simulink model "large_scale_autosar_swc_expfcns"  (R2021a)
settings: Solver=FixedStepDiscrete  StartTime=0.0  StopTime=20  FixedStep=1  MaxStep=.0001  RelTol=1e-3  EnableMultiTasking=on
undefined symbols (not defined in the file): DiscIntNeverNeededParam
(part 1 of 3)
settings Model: ExtModeAutoUpdateStatusClock=off  Creator=The MathWorks, Inc.  LastModifiedBy=ASUS
settings SolverCC: AlgebraicLoopSolver=TrustRegion
settings DataIOCC: LimitDataPoints=on  SaveFormat=Array  SaveOutput=off  SaveTime=off  ReturnWorkspaceOutputs=off
settings OptimizationCC: DefaultParameterBehavior=Inlined  InlineInvariantSignals=on  EnhancedBackFolding=on  ExpressionDepthLimit=2147483647  StateBitsets=on  DataBitsets=on  ZeroExternalMemoryAtStartup=off  ZeroInternalMemoryAtStartup=off  NoFixptDivByZeroProtection=on  EfficientFloat2IntCast=on  EfficientMapNaN2IntZero=off  LifeSpan=1  BufferReusableBoundary=off  EfficientTunableParamExpr=on
settings DebuggingCC: SigSpecEnsureSampleTimeMsg=none  BusObjectLabelMismatch=none  AllowSymbolicDim=off  StateNameClashWarn=warning  PregeneratedLibrarySubsystemCodeDiagnostic=none  StrictBusMsg=ErrorOnBusTreatedAsVector  SFUnexpectedBacktrackingDiag=warning  SFNoUnconditionalDefaultTransitionDiag=warning  SFExecutionAtInitializationDiag=none  SFMachineParentedDataDiag=warning  ArithmeticOperatorsInVariantConditions=warning
settings HardwareCC: ProdLongLongMode=on  TargetIntDivRoundTo=Zero  TargetEndianess=LittleEndian  TargetHWDeviceType=Generic->32-bit Embedded Processor
settings ModelReferenceCC: ModelReferenceNumInstancesAllowed=Single  PropagateSignalLabelsOutOfModel=off
settings SFSimCC: SimUseLocalCustomCode=off  SimParseCustomCode=off  CustomCodeUndefinedFunction=UseInterfaceOnly
settings RTWCC: Description=AUTOSAR  SystemTargetFile=autosar.tlc  GenCodeOnly=on  TemplateMakefile=ert_default_tmf  GenerateReport=on  RTWVerbose=off  RTWUseLocalCustomCode=off  IncludeHyperlinkInReport=on  LaunchReport=on  PortableWordSizes=on
settings CodeAppCC: ForceParamTrailComments=on  IgnoreCustomStorageClasses=off  IgnoreTestpoints=on  SimulinkDataObjDesc=on  CustomSymbolStrGlobalVar=rt$N$M  CustomSymbolStrType=$N$M  CustomSymbolStrFcn=$N$M$F  CustomSymbolStrMacro=$N$M  InsertBlockDesc=on  StateflowObjectComments=on  InternalIdentifier=Classic
settings STFCustomTargetCC: UtilityFuncGeneration=Shared location  ParMdlRefBuildCompliant=on  CompOptLevelCompliant=on  IncludeMdlTerminateFcn=off  CombineOutputUpdateFcns=on  SuppressErrorStatus=on  ERTCustomFileBanners=on  SupportNonFinite=off  SupportComplex=off  SupportContinuousTime=off  SupportNonInlinedSFcns=off  RemoveResetFunc=on  MATLABClassNameForMDSCustomization=Simulink.SoftwareTarget.ERTCustomization  CPPClassGenCompliant=on  AutosarCompliant=on  GRTInterface=off  LookupTableObjectStructAxisOrder=2,1,3,4,...  LUTObjectStructOrderEvenSpacing=Size,Table,Breakpoints  SystemTargetFile=autosar.tlc
settings ERTTargetCC: UtilityFuncGeneration=Shared location  MultiwordLength=2048  ConcurrentExecutionCompliant=off  IncludeMdlTerminateFcn=off  SuppressErrorStatus=on  SupportNonFinite=off  SupportComplex=off  ModelStepFunctionPrototypeControlCompliant=off  AutosarCompliant=on  LookupTableObjectStructAxisOrder=2,1,3,4,...  LUTObjectStructOrderEvenSpacing=Size,Table,Breakpoints  ExtModeMexFile=noextcomm  InlinedParameterPlacement=NonHierarchical  ERTCustomFileTemplate=example_file_process.tlc  ERTFilePackagingFormat=CompactWithDataFile  ConvertIfToSwitch=off  SuppressUnreachableDefaultCases=off
settings ConfigComp: CovMetricSettings=dw  CovSaveCumulativeToWorkspaceVar=on  CovSaveSingleToWorkspaceVar=on  CovExternalEMLEnable=off

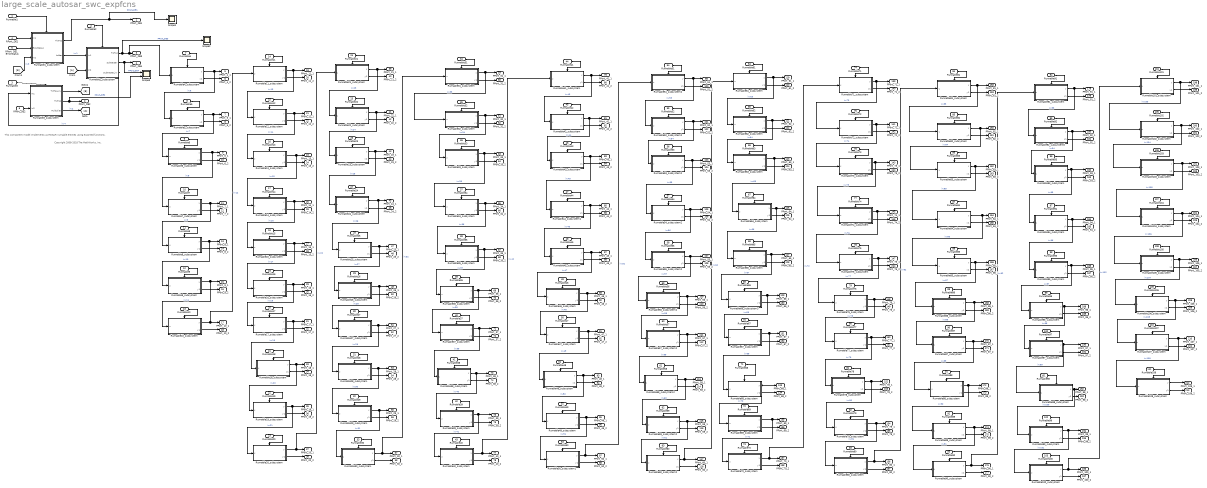
== system large_scale_autosar_swc_expfcns ==
  note: This component model implements AUTOSAR runnable entities using exported functions.
  note: Copyright 2008-2018 The MathWorks, Inc.
  Runnable1 : Inport  PortDimensions=1  SampleTime=1  OutputFunctionCall=on
  Runnable2 : Inport  Port=2  PortDimensions=1  SampleTime=1  OutputFunctionCall=on
  Runnable3 : Inport  Port=3  PortDimensions=1  SampleTime=10  OutputFunctionCall=on
  RPort_DE1 : Inport  Port=4  OutDataTypeStr=double  PortDimensions=1
  RPort_DE1_ErrorStatus : Inport  Port=5  OutDataTypeStr=uint8  PortDimensions=1
  RPort_DE2 : Inport  Port=6  OutDataTypeStr=double  PortDimensions=2
  Runnable4 : Inport  Port=7  PortDimensions=1  SampleTime=1  OutputFunctionCall=on
  Runnable5 : Inport  Port=8  PortDimensions=1  SampleTime=1  OutputFunctionCall=on
  Runnable6 : Inport  Port=9  PortDimensions=1  SampleTime=1  OutputFunctionCall=on
  Runnable7 : Inport  Port=10  PortDimensions=1  SampleTime=1  OutputFunctionCall=on
  Runnable8 : Inport  Port=11  PortDimensions=1  SampleTime=1  OutputFunctionCall=on
  Runnable9 : Inport  Port=12  PortDimensions=1  SampleTime=1  OutputFunctionCall=on
  Runnable10 : Inport  Port=13  PortDimensions=1  SampleTime=1  OutputFunctionCall=on
  Runnable11 : Inport  Port=14  PortDimensions=1  SampleTime=1  OutputFunctionCall=on
  Runnable12 : Inport  Port=15  PortDimensions=1  SampleTime=1  OutputFunctionCall=on
  Runnable13 : Inport  Port=16  PortDimensions=1  SampleTime=1  OutputFunctionCall=on
  Runnable14 : Inport  Port=17  PortDimensions=1  SampleTime=1  OutputFunctionCall=on
  Runnable15 : Inport  Port=18  PortDimensions=1  SampleTime=1  OutputFunctionCall=on
  Runnable16 : Inport  Port=19  PortDimensions=1  SampleTime=1  OutputFunctionCall=on
  Runnable17 : Inport  Port=20  PortDimensions=1  SampleTime=1  OutputFunctionCall=on
  Runnable18 : Inport  Port=21  PortDimensions=1  SampleTime=1  OutputFunctionCall=on
  Runnable19 : Inport  Port=22  PortDimensions=1  SampleTime=1  OutputFunctionCall=on
  Runnable20 : Inport  Port=23  PortDimensions=1  SampleTime=1  OutputFunctionCall=on
  Runnable21 : Inport  Port=24  PortDimensions=1  SampleTime=1  OutputFunctionCall=on
  Runnable22 : Inport  Port=25  PortDimensions=1  SampleTime=1  OutputFunctionCall=on
  Runnable23 : Inport  Port=26  PortDimensions=1  SampleTime=1  OutputFunctionCall=on
  Runnable24 : Inport  Port=27  PortDimensions=1  SampleTime=1  OutputFunctionCall=on
  Runnable25 : Inport  Port=28  PortDimensions=1  SampleTime=1  OutputFunctionCall=on
  Runnable26 : Inport  Port=29  PortDimensions=1  SampleTime=1  OutputFunctionCall=on
  Runnable27 : Inport  Port=30  PortDimensions=1  SampleTime=1  OutputFunctionCall=on
  Runnable28 : Inport  Port=31  PortDimensions=1  SampleTime=1  OutputFunctionCall=on
  Runnable29 : Inport  Port=32  PortDimensions=1  SampleTime=1  OutputFunctionCall=on
  Runnable30 : Inport  Port=33  PortDimensions=1  SampleTime=1  OutputFunctionCall=on
  Runnable31 : Inport  Port=34  PortDimensions=1  SampleTime=1  OutputFunctionCall=on
  Runnable32 : Inport  Port=35  PortDimensions=1  SampleTime=1  OutputFunctionCall=on
  Runnable33 : Inport  Port=36  PortDimensions=1  SampleTime=1  OutputFunctionCall=on
  Runnable34 : Inport  Port=37  PortDimensions=1  SampleTime=1  OutputFunctionCall=on
  Runnable35 : Inport  Port=38  PortDimensions=1  SampleTime=1  OutputFunctionCall=on
  Runnable36 : Inport  Port=39  PortDimensions=1  SampleTime=1  OutputFunctionCall=on
  Runnable37 : Inport  Port=40  PortDimensions=1  SampleTime=1  OutputFunctionCall=on
  Runnable38 : Inport  Port=41  PortDimensions=1  SampleTime=1  OutputFunctionCall=on
  Runnable39 : Inport  Port=42  PortDimensions=1  SampleTime=1  OutputFunctionCall=on
  Runnable40 : Inport  Port=43  PortDimensions=1  SampleTime=1  OutputFunctionCall=on
  Runnable41 : Inport  Port=44  PortDimensions=1  SampleTime=1  OutputFunctionCall=on
  Runnable42 : Inport  Port=45  PortDimensions=1  SampleTime=1  OutputFunctionCall=on
  Runnable43 : Inport  Port=46  PortDimensions=1  SampleTime=1  OutputFunctionCall=on
  Runnable44 : Inport  Port=47  PortDimensions=1  SampleTime=1  OutputFunctionCall=on
  Runnable45 : Inport  Port=48  PortDimensions=1  SampleTime=1  OutputFunctionCall=on
  Runnable46 : Inport  Port=49  PortDimensions=1  SampleTime=1  OutputFunctionCall=on
  Runnable47 : Inport  Port=50  PortDimensions=1  SampleTime=1  OutputFunctionCall=on
  Runnable48 : Inport  Port=51  PortDimensions=1  SampleTime=1  OutputFunctionCall=on
  Runnable49 : Inport  Port=52  PortDimensions=1  SampleTime=1  OutputFunctionCall=on
  Runnable50 : Inport  Port=53  PortDimensions=1  SampleTime=1  OutputFunctionCall=on
  Runnable51 : Inport  Port=54  PortDimensions=1  SampleTime=1  OutputFunctionCall=on
  Runnable52 : Inport  Port=55  PortDimensions=1  SampleTime=1  OutputFunctionCall=on
  Runnable53 : Inport  Port=56  PortDimensions=1  SampleTime=1  OutputFunctionCall=on
  Runnable54 : Inport  Port=57  PortDimensions=1  SampleTime=1  OutputFunctionCall=on
  Runnable55 : Inport  Port=58  PortDimensions=1  SampleTime=1  OutputFunctionCall=on
  Runnable56 : Inport  Port=59  PortDimensions=1  SampleTime=1  OutputFunctionCall=on
  Runnable57 : Inport  Port=60  PortDimensions=1  SampleTime=1  OutputFunctionCall=on
  Runnable58 : Inport  Port=61  PortDimensions=1  SampleTime=1  OutputFunctionCall=on
  Runnable59 : Inport  Port=62  PortDimensions=1  SampleTime=1  OutputFunctionCall=on
  Runnable60 : Inport  Port=63  PortDimensions=1  SampleTime=1  OutputFunctionCall=on
  Runnable61 : Inport  Port=64  PortDimensions=1  SampleTime=1  OutputFunctionCall=on
  Runnable62 : Inport  Port=65  PortDimensions=1  SampleTime=1  OutputFunctionCall=on
  Runnable63 : Inport  Port=66  PortDimensions=1  SampleTime=1  OutputFunctionCall=on
  Runnable64 : Inport  Port=67  PortDimensions=1  SampleTime=1  OutputFunctionCall=on
  Runnable65 : Inport  Port=68  PortDimensions=1  SampleTime=1  OutputFunctionCall=on
  Runnable66 : Inport  Port=69  PortDimensions=1  SampleTime=1  OutputFunctionCall=on
  Runnable67 : Inport  Port=70  PortDimensions=1  SampleTime=1  OutputFunctionCall=on
  Runnable68 : Inport  Port=71  PortDimensions=1  SampleTime=1  OutputFunctionCall=on
  Runnable69 : Inport  Port=72  PortDimensions=1  SampleTime=1  OutputFunctionCall=on
  Runnable70 : Inport  Port=73  PortDimensions=1  SampleTime=1  OutputFunctionCall=on
  Runnable71 : Inport  Port=74  PortDimensions=1  SampleTime=1  OutputFunctionCall=on
  Runnable72 : Inport  Port=75  PortDimensions=1  SampleTime=1  OutputFunctionCall=on
  Runnable73 : Inport  Port=76  PortDimensions=1  SampleTime=1  OutputFunctionCall=on
  Runnable74 : Inport  Port=77  PortDimensions=1  SampleTime=1  OutputFunctionCall=on
  Runnable75 : Inport  Port=78  PortDimensions=1  SampleTime=1  OutputFunctionCall=on
  Runnable76 : Inport  Port=79  PortDimensions=1  SampleTime=1  OutputFunctionCall=on
  Runnable77 : Inport  Port=80  PortDimensions=1  SampleTime=1  OutputFunctionCall=on
  Runnable78 : Inport  Port=81  PortDimensions=1  SampleTime=1  OutputFunctionCall=on
  Runnable79 : Inport  Port=82  PortDimensions=1  SampleTime=1  OutputFunctionCall=on
  Runnable80 : Inport  Port=83  PortDimensions=1  SampleTime=1  OutputFunctionCall=on
  Runnable81 : Inport  Port=84  PortDimensions=1  SampleTime=1  OutputFunctionCall=on
  Runnable82 : Inport  Port=85  PortDimensions=1  SampleTime=1  OutputFunctionCall=on
  Runnable83 : Inport  Port=86  PortDimensions=1  SampleTime=1  OutputFunctionCall=on
  Runnable84 : Inport  Port=87  PortDimensions=1  SampleTime=1  OutputFunctionCall=on
  Runnable85 : Inport  Port=88  PortDimensions=1  SampleTime=1  OutputFunctionCall=on
  Runnable86 : Inport  Port=89  PortDimensions=1  SampleTime=1  OutputFunctionCall=on
  Runnable87 : Inport  Port=90  PortDimensions=1  SampleTime=1  OutputFunctionCall=on
  Runnable88 : Inport  Port=91  PortDimensions=1  SampleTime=1  OutputFunctionCall=on
  Runnable89 : Inport  Port=92  PortDimensions=1  SampleTime=1  OutputFunctionCall=on
  Runnable90 : Inport  Port=93  PortDimensions=1  SampleTime=1  OutputFunctionCall=on
  Runnable91 : Inport  Port=94  PortDimensions=1  SampleTime=1  OutputFunctionCall=on
  Runnable92 : Inport  Port=95  PortDimensions=1  SampleTime=1  OutputFunctionCall=on
  Runnable93 : Inport  Port=96  PortDimensions=1  SampleTime=1  OutputFunctionCall=on
  Runnable94 : Inport  Port=97  PortDimensions=1  SampleTime=1  OutputFunctionCall=on
  Runnable95 : Inport  Port=98  PortDimensions=1  SampleTime=1  OutputFunctionCall=on
  Runnable96 : Inport  Port=99  PortDimensions=1  SampleTime=1  OutputFunctionCall=on
  Runnable97 : Inport  Port=100  PortDimensions=1  SampleTime=1  OutputFunctionCall=on
  Runnable98 : Inport  Port=101  PortDimensions=1  SampleTime=1  OutputFunctionCall=on
  Runnable99 : Inport  Port=102  PortDimensions=1  SampleTime=1  OutputFunctionCall=on
  Runnable100 : Inport  Port=103  PortDimensions=1  SampleTime=1  OutputFunctionCall=on
  Runnable101 : Inport  Port=104  PortDimensions=1  SampleTime=1  OutputFunctionCall=on
  Runnable102 : Inport  Port=105  PortDimensions=1  SampleTime=1  OutputFunctionCall=on
  Runnable103 : Inport  Port=106  PortDimensions=1  SampleTime=1  OutputFunctionCall=on
  Runnable104 : Inport  Port=107  PortDimensions=1  SampleTime=1  OutputFunctionCall=on
  Runnable105 : Inport  Port=108  PortDimensions=1  SampleTime=1  OutputFunctionCall=on
  Runnable106 : Inport  Port=109  PortDimensions=1  SampleTime=1  OutputFunctionCall=on
  Runnable107 : Inport  Port=110  PortDimensions=1  SampleTime=1  OutputFunctionCall=on
  Runnable108 : Inport  Port=111  PortDimensions=1  SampleTime=1  OutputFunctionCall=on
  Runnable100_subsystem : Subsystem  TreatAsAtomicUnit=on  RTWFcnName=foo
  Runnable101_subsystem : Subsystem  TreatAsAtomicUnit=on  RTWFcnName=foo
  Runnable102_subsystem : Subsystem  TreatAsAtomicUnit=on  RTWFcnName=foo
  Runnable103_subsystem : Subsystem  TreatAsAtomicUnit=on  RTWFcnName=foo
  Runnable104_subsystem : Subsystem  TreatAsAtomicUnit=on  RTWFcnName=foo
  Runnable105_subsystem : Subsystem  TreatAsAtomicUnit=on  RTWFcnName=foo
  Runnable106_subsystem : Subsystem  TreatAsAtomicUnit=on  RTWFcnName=foo
  Runnable107_subsystem : Subsystem  TreatAsAtomicUnit=on  RTWFcnName=foo
  Runnable108_subsystem : Subsystem  TreatAsAtomicUnit=on  RTWFcnName=foo
  Runnable10_subsystem : Subsystem  TreatAsAtomicUnit=on  RTWFcnName=foo
  Runnable11_subsystem : Subsystem  TreatAsAtomicUnit=on  RTWFcnName=foo
  Runnable12_subsystem : Subsystem  TreatAsAtomicUnit=on  RTWFcnName=foo
  Runnable13_subsystem : Subsystem  TreatAsAtomicUnit=on  RTWFcnName=foo
  Runnable14_subsystem : Subsystem  TreatAsAtomicUnit=on  RTWFcnName=foo
  Runnable15_subsystem : Subsystem  TreatAsAtomicUnit=on  RTWFcnName=foo
  Runnable16_subsystem : Subsystem  TreatAsAtomicUnit=on  RTWFcnName=foo
  Runnable17_subsystem : Subsystem  TreatAsAtomicUnit=on  RTWFcnName=foo
  Runnable18_subsystem : Subsystem  TreatAsAtomicUnit=on  RTWFcnName=foo
  Runnable19_subsystem : Subsystem  TreatAsAtomicUnit=on  RTWFcnName=foo
  Runnable1_subsystem : Subsystem  TreatAsAtomicUnit=on  RTWFcnName=foo
  Runnable20_subsystem : Subsystem  TreatAsAtomicUnit=on  RTWFcnName=foo
  Runnable21_subsystem : Subsystem  TreatAsAtomicUnit=on  RTWFcnName=foo
  Runnable22_subsystem : Subsystem  TreatAsAtomicUnit=on  RTWFcnName=foo
  Runnable23_subsystem : Subsystem  TreatAsAtomicUnit=on  RTWFcnName=foo
  Runnable24_subsystem : Subsystem  TreatAsAtomicUnit=on  RTWFcnName=foo
  Runnable25_subsystem : Subsystem  TreatAsAtomicUnit=on  RTWFcnName=foo
  Runnable26_subsystem : Subsystem  TreatAsAtomicUnit=on  RTWFcnName=foo
  Runnable27_subsystem : Subsystem  TreatAsAtomicUnit=on  RTWFcnName=foo
  Runnable28_subsystem : Subsystem  TreatAsAtomicUnit=on  RTWFcnName=foo
  Runnable29_subsystem : Subsystem  TreatAsAtomicUnit=on  RTWFcnName=foo
  Runnable2_subsystem : Subsystem  TreatAsAtomicUnit=on  RTWFcnName=foo
  Runnable30_subsystem : Subsystem  TreatAsAtomicUnit=on  RTWFcnName=foo
  Runnable31_subsystem : Subsystem  TreatAsAtomicUnit=on  RTWFcnName=foo
  Runnable32_subsystem : Subsystem  TreatAsAtomicUnit=on  RTWFcnName=foo
  Runnable33_subsystem : Subsystem  TreatAsAtomicUnit=on  RTWFcnName=foo
  Runnable34_subsystem : Subsystem  TreatAsAtomicUnit=on  RTWFcnName=foo
  Runnable35_subsystem : Subsystem  TreatAsAtomicUnit=on  RTWFcnName=foo
  Runnable36_subsystem : Subsystem  TreatAsAtomicUnit=on  RTWFcnName=foo
  Runnable37_subsystem : Subsystem  TreatAsAtomicUnit=on  RTWFcnName=foo
  Runnable38_subsystem : Subsystem  TreatAsAtomicUnit=on  RTWFcnName=foo
  Runnable39_subsystem : Subsystem  TreatAsAtomicUnit=on  RTWFcnName=foo
  Runnable3_subsystem : Subsystem  TreatAsAtomicUnit=on  RTWFcnName=foo
  Runnable40_subsystem : Subsystem  TreatAsAtomicUnit=on  RTWFcnName=foo
  Runnable41_subsystem : Subsystem  TreatAsAtomicUnit=on  RTWFcnName=foo
  Runnable42_subsystem : Subsystem  TreatAsAtomicUnit=on  RTWFcnName=foo
  Runnable43_subsystem : Subsystem  TreatAsAtomicUnit=on  RTWFcnName=foo
  Runnable44_subsystem1 : Subsystem  TreatAsAtomicUnit=on  RTWFcnName=foo
  Runnable45_subsystem : Subsystem  TreatAsAtomicUnit=on  RTWFcnName=foo
  Runnable46_subsystem : Subsystem  TreatAsAtomicUnit=on  RTWFcnName=foo
  Runnable47_subsystem : Subsystem  TreatAsAtomicUnit=on  RTWFcnName=foo
  Runnable48_subsystem : Subsystem  TreatAsAtomicUnit=on  RTWFcnName=foo
  Runnable49_subsystem : Subsystem  TreatAsAtomicUnit=on  RTWFcnName=foo
  Runnable4_subsystem : Subsystem  TreatAsAtomicUnit=on  RTWFcnName=foo
  Runnable50_subsystem1 : Subsystem  TreatAsAtomicUnit=on  RTWFcnName=foo
  Runnable51_subsystem2 : Subsystem  TreatAsAtomicUnit=on  RTWFcnName=foo
  Runnable52_subsystem2 : Subsystem  TreatAsAtomicUnit=on  RTWFcnName=foo
  Runnable53_subsystem2 : Subsystem  TreatAsAtomicUnit=on  RTWFcnName=foo
  Runnable54_subsystem2 : Subsystem  TreatAsAtomicUnit=on  RTWFcnName=foo
  Runnable55_subsystem2 : Subsystem  TreatAsAtomicUnit=on  RTWFcnName=foo
  Runnable56_subsystem2 : Subsystem  TreatAsAtomicUnit=on  RTWFcnName=foo
  Runnable57_subsystem2 : Subsystem  TreatAsAtomicUnit=on  RTWFcnName=foo
  Runnable58_subsystem2 : Subsystem  TreatAsAtomicUnit=on  RTWFcnName=foo
  Runnable59_subsystem2 : Subsystem  TreatAsAtomicUnit=on  RTWFcnName=foo
  Runnable5_subsystem : Subsystem  TreatAsAtomicUnit=on  RTWFcnName=foo
  Runnable60_subsystem2 : Subsystem  TreatAsAtomicUnit=on  RTWFcnName=foo
  Runnable61_subsystem : Subsystem  TreatAsAtomicUnit=on  RTWFcnName=foo
  Runnable62_subsystem : Subsystem  TreatAsAtomicUnit=on  RTWFcnName=foo
  Runnable63_subsystem : Subsystem  TreatAsAtomicUnit=on  RTWFcnName=foo
  Runnable64_subsystem : Subsystem  TreatAsAtomicUnit=on  RTWFcnName=foo
  Runnable65_subsystem : Subsystem  TreatAsAtomicUnit=on  RTWFcnName=foo
  Runnable66_subsystem3 : Subsystem  TreatAsAtomicUnit=on  RTWFcnName=foo
  Runnable67_subsystem : Subsystem  TreatAsAtomicUnit=on  RTWFcnName=foo
  Runnable68_subsystem : Subsystem  TreatAsAtomicUnit=on  RTWFcnName=foo
  Runnable69_subsystem : Subsystem  TreatAsAtomicUnit=on  RTWFcnName=foo
  Runnable6_subsystem : Subsystem  TreatAsAtomicUnit=on  RTWFcnName=foo
  Runnable70_subsystem : Subsystem  TreatAsAtomicUnit=on  RTWFcnName=foo
  Runnable71_subsystem : Subsystem  TreatAsAtomicUnit=on  RTWFcnName=foo
  Runnable72_subsystem : Subsystem  TreatAsAtomicUnit=on  RTWFcnName=foo
  Runnable73_subsystem : Subsystem  TreatAsAtomicUnit=on  RTWFcnName=foo
  Runnable74_subsystem : Subsystem  TreatAsAtomicUnit=on  RTWFcnName=foo
  Runnable75_subsystem : Subsystem  TreatAsAtomicUnit=on  RTWFcnName=foo
  Runnable76_subsystem : Subsystem  TreatAsAtomicUnit=on  RTWFcnName=foo
  Runnable77_subsystem : Subsystem  TreatAsAtomicUnit=on  RTWFcnName=foo
  Runnable78_subsystem : Subsystem  TreatAsAtomicUnit=on  RTWFcnName=foo
  Runnable79_subsystem : Subsystem  TreatAsAtomicUnit=on  RTWFcnName=foo
  Runnable7_subsystem : Subsystem  TreatAsAtomicUnit=on  RTWFcnName=foo
  Runnable80_subsystem : Subsystem  TreatAsAtomicUnit=on  RTWFcnName=foo
  Runnable81_subsystem : Subsystem  TreatAsAtomicUnit=on  RTWFcnName=foo
  Runnable82_subsystem : Subsystem  TreatAsAtomicUnit=on  RTWFcnName=foo
  Runnable83_subsystem : Subsystem  TreatAsAtomicUnit=on  RTWFcnName=foo
  Runnable84_subsystem : Subsystem  TreatAsAtomicUnit=on  RTWFcnName=foo
  Runnable85_subsystem : Subsystem  TreatAsAtomicUnit=on  RTWFcnName=foo
  Runnable86_subsystem : Subsystem  TreatAsAtomicUnit=on  RTWFcnName=foo
  Runnable87_subsystem : Subsystem  TreatAsAtomicUnit=on  RTWFcnName=foo
  Runnable88_subsystem : Subsystem  TreatAsAtomicUnit=on  RTWFcnName=foo
  Runnable89_subsystem : Subsystem  TreatAsAtomicUnit=on  RTWFcnName=foo
  Runnable8_subsystem : Subsystem  TreatAsAtomicUnit=on  RTWFcnName=foo
  Runnable90_subsystem : Subsystem  TreatAsAtomicUnit=on  RTWFcnName=foo
  Runnable91_subsystem : Subsystem  TreatAsAtomicUnit=on  RTWFcnName=foo
  Runnable92_subsystem6 : Subsystem  TreatAsAtomicUnit=on  RTWFcnName=foo
  Runnable93_subsystem : Subsystem  TreatAsAtomicUnit=on  RTWFcnName=foo
  Runnable94_subsystem : Subsystem  TreatAsAtomicUnit=on  RTWFcnName=foo
  Runnable95_subsystem : Subsystem  TreatAsAtomicUnit=on  RTWFcnName=foo
  Runnable96_subsystem : Subsystem  TreatAsAtomicUnit=on  RTWFcnName=foo
  Runnable97_subsystem : Subsystem  TreatAsAtomicUnit=on  RTWFcnName=foo
  Runnable98_subsystem : Subsystem  TreatAsAtomicUnit=on  RTWFcnName=foo
  Runnable99_subsystem : Subsystem  TreatAsAtomicUnit=on  RTWFcnName=foo
  Runnable9_subsystem : Subsystem  TreatAsAtomicUnit=on  RTWFcnName=foo
  Scope1 : Scope
  Scope2 : Scope
  Scope3 : Scope  NumInputPorts=2
  PPort_DE1 : Outport  OutDataTypeStr=int8  PortDimensions=1  VectorParamsAs1DForOutWhenUnconnected=off
  PPort_DE2 : Outport  Port=2  OutDataTypeStr=int8  PortDimensions=1  VectorParamsAs1DForOutWhenUnconnected=off
  PPort_DE3 : Outport  Port=3  OutDataTypeStr=int8  PortDimensions=2  VectorParamsAs1DForOutWhenUnconnected=off
  PPort_DE4 : Outport  Port=4  OutDataTypeStr=double  PortDimensions=1  VectorParamsAs1DForOutWhenUnconnected=off
  PPort_4_1 : Outport  Port=5  OutDataTypeStr=int8  PortDimensions=2  VectorParamsAs1DForOutWhenUnconnected=off
  PPort_4_2 : Outport  Port=6  OutDataTypeStr=int8  PortDimensions=2  VectorParamsAs1DForOutWhenUnconnected=off
  PPort_5_1 : Outport  Port=7  OutDataTypeStr=int8  PortDimensions=2  VectorParamsAs1DForOutWhenUnconnected=off
  PPort_5_2 : Outport  Port=8  OutDataTypeStr=int8  PortDimensions=2  VectorParamsAs1DForOutWhenUnconnected=off
  PPort_6_1 : Outport  Port=9  OutDataTypeStr=int8  PortDimensions=2  VectorParamsAs1DForOutWhenUnconnected=off
  PPort_6_2 : Outport  Port=10  OutDataTypeStr=int8  PortDimensions=2  VectorParamsAs1DForOutWhenUnconnected=off
  PPort_7_1 : Outport  Port=11  OutDataTypeStr=int8  PortDimensions=2  VectorParamsAs1DForOutWhenUnconnected=off
  PPort_7_2 : Outport  Port=12  OutDataTypeStr=int8  PortDimensions=2  VectorParamsAs1DForOutWhenUnconnected=off
  PPort_8_1 : Outport  Port=13  OutDataTypeStr=int8  PortDimensions=2  VectorParamsAs1DForOutWhenUnconnected=off
  PPort_8_2 : Outport  Port=14  OutDataTypeStr=int8  PortDimensions=2  VectorParamsAs1DForOutWhenUnconnected=off
  PPort_9_1 : Outport  Port=15  OutDataTypeStr=int8  PortDimensions=2  VectorParamsAs1DForOutWhenUnconnected=off
  PPort_9_2 : Outport  Port=16  OutDataTypeStr=int8  PortDimensions=2  VectorParamsAs1DForOutWhenUnconnected=off
  PPort_10_1 : Outport  Port=17  OutDataTypeStr=int8  PortDimensions=2  VectorParamsAs1DForOutWhenUnconnected=off
  PPort_10_2 : Outport  Port=18  OutDataTypeStr=int8  PortDimensions=2  VectorParamsAs1DForOutWhenUnconnected=off
  PPort_11_1 : Outport  Port=19  OutDataTypeStr=int8  PortDimensions=2  VectorParamsAs1DForOutWhenUnconnected=off
  PPort_11_2 : Outport  Port=20  OutDataTypeStr=int8  PortDimensions=2  VectorParamsAs1DForOutWhenUnconnected=off
  PPort_12_1 : Outport  Port=21  OutDataTypeStr=int8  PortDimensions=2  VectorParamsAs1DForOutWhenUnconnected=off
  PPort_12_2 : Outport  Port=22  OutDataTypeStr=int8  PortDimensions=2  VectorParamsAs1DForOutWhenUnconnected=off
  PPort_13_1 : Outport  Port=23  OutDataTypeStr=int8  PortDimensions=2  VectorParamsAs1DForOutWhenUnconnected=off
  PPort_13_2 : Outport  Port=24  OutDataTypeStr=int8  PortDimensions=2  VectorParamsAs1DForOutWhenUnconnected=off
  PPort_14_1 : Outport  Port=25  OutDataTypeStr=int8  PortDimensions=2  VectorParamsAs1DForOutWhenUnconnected=off
  PPort_14_2 : Outport  Port=26  OutDataTypeStr=int8  PortDimensions=2  VectorParamsAs1DForOutWhenUnconnected=off
  PPort_15_1 : Outport  Port=27  OutDataTypeStr=int8  PortDimensions=2  VectorParamsAs1DForOutWhenUnconnected=off
  PPort_15_2 : Outport  Port=28  OutDataTypeStr=int8  PortDimensions=2  VectorParamsAs1DForOutWhenUnconnected=off
  PPort_16_1 : Outport  Port=29  OutDataTypeStr=int8  PortDimensions=2  VectorParamsAs1DForOutWhenUnconnected=off
  PPort_16_2 : Outport  Port=30  OutDataTypeStr=int8  PortDimensions=2  VectorParamsAs1DForOutWhenUnconnected=off
  PPort_17_1 : Outport  Port=31  OutDataTypeStr=int8  PortDimensions=2  VectorParamsAs1DForOutWhenUnconnected=off
  PPort_17_2 : Outport  Port=32  OutDataTypeStr=int8  PortDimensions=2  VectorParamsAs1DForOutWhenUnconnected=off
  PPort_18_1 : Outport  Port=33  OutDataTypeStr=int8  PortDimensions=2  VectorParamsAs1DForOutWhenUnconnected=off
  PPort_18_2 : Outport  Port=34  OutDataTypeStr=int8  PortDimensions=2  VectorParamsAs1DForOutWhenUnconnected=off
  PPort_19_1 : Outport  Port=35  OutDataTypeStr=int8  PortDimensions=2  VectorParamsAs1DForOutWhenUnconnected=off
  PPort_19_2 : Outport  Port=36  OutDataTypeStr=int8  PortDimensions=2  VectorParamsAs1DForOutWhenUnconnected=off
  PPort_20_1 : Outport  Port=37  OutDataTypeStr=int8  PortDimensions=2  VectorParamsAs1DForOutWhenUnconnected=off
  PPort_20_2 : Outport  Port=38  OutDataTypeStr=int8  PortDimensions=2  VectorParamsAs1DForOutWhenUnconnected=off
  PPort_21_1 : Outport  Port=39  OutDataTypeStr=int8  PortDimensions=2  VectorParamsAs1DForOutWhenUnconnected=off
  PPort_21_2 : Outport  Port=40  OutDataTypeStr=int8  PortDimensions=2  VectorParamsAs1DForOutWhenUnconnected=off
  PPort_22_1 : Outport  Port=41  OutDataTypeStr=int8  PortDimensions=2  VectorParamsAs1DForOutWhenUnconnected=off
  PPort_22_2 : Outport  Port=42  OutDataTypeStr=int8  PortDimensions=2  VectorParamsAs1DForOutWhenUnconnected=off
  PPort_23_1 : Outport  Port=43  OutDataTypeStr=int8  PortDimensions=2  VectorParamsAs1DForOutWhenUnconnected=off
  PPort_23_2 : Outport  Port=44  OutDataTypeStr=int8  PortDimensions=2  VectorParamsAs1DForOutWhenUnconnected=off
  PPort_24_1 : Outport  Port=45  OutDataTypeStr=int8  PortDimensions=2  VectorParamsAs1DForOutWhenUnconnected=off
  PPort_24_2 : Outport  Port=46  OutDataTypeStr=int8  PortDimensions=2  VectorParamsAs1DForOutWhenUnconnected=off
  PPort_25_1 : Outport  Port=47  OutDataTypeStr=int8  PortDimensions=2  VectorParamsAs1DForOutWhenUnconnected=off
  PPort_25_2 : Outport  Port=48  OutDataTypeStr=int8  PortDimensions=2  VectorParamsAs1DForOutWhenUnconnected=off
  PPort_26_1 : Outport  Port=49  OutDataTypeStr=int8  PortDimensions=2  VectorParamsAs1DForOutWhenUnconnected=off
  PPort_26_2 : Outport  Port=50  OutDataTypeStr=int8  PortDimensions=2  VectorParamsAs1DForOutWhenUnconnected=off
  PPort_27_1 : Outport  Port=51  OutDataTypeStr=int8  PortDimensions=2  VectorParamsAs1DForOutWhenUnconnected=off
  PPort_27_2 : Outport  Port=52  OutDataTypeStr=int8  PortDimensions=2  VectorParamsAs1DForOutWhenUnconnected=off
  PPort_28_1 : Outport  Port=53  OutDataTypeStr=int8  PortDimensions=2  VectorParamsAs1DForOutWhenUnconnected=off
  PPort_28_2 : Outport  Port=54  OutDataTypeStr=int8  PortDimensions=2  VectorParamsAs1DForOutWhenUnconnected=off
  PPort_29_1 : Outport  Port=55  OutDataTypeStr=int8  PortDimensions=2  VectorParamsAs1DForOutWhenUnconnected=off
  PPort_29_2 : Outport  Port=56  OutDataTypeStr=int8  PortDimensions=2  VectorParamsAs1DForOutWhenUnconnected=off
  PPort_30_1 : Outport  Port=57  OutDataTypeStr=int8  PortDimensions=2  VectorParamsAs1DForOutWhenUnconnected=off
  PPort_30_2 : Outport  Port=58  OutDataTypeStr=int8  PortDimensions=2  VectorParamsAs1DForOutWhenUnconnected=off
  PPort_31_1 : Outport  Port=59  OutDataTypeStr=int8  PortDimensions=2  VectorParamsAs1DForOutWhenUnconnected=off
  PPort_31_2 : Outport  Port=60  OutDataTypeStr=int8  PortDimensions=2  VectorParamsAs1DForOutWhenUnconnected=off
  PPort_32_1 : Outport  Port=61  OutDataTypeStr=int8  PortDimensions=2  VectorParamsAs1DForOutWhenUnconnected=off
  PPort_32_2 : Outport  Port=62  OutDataTypeStr=int8  PortDimensions=2  VectorParamsAs1DForOutWhenUnconnected=off
  PPort_33_1 : Outport  Port=63  OutDataTypeStr=int8  PortDimensions=2  VectorParamsAs1DForOutWhenUnconnected=off
  PPort_33_2 : Outport  Port=64  OutDataTypeStr=int8  PortDimensions=2  VectorParamsAs1DForOutWhenUnconnected=off
  PPort_34_1 : Outport  Port=65  OutDataTypeStr=int8  PortDimensions=2  VectorParamsAs1DForOutWhenUnconnected=off
  PPort_34_2 : Outport  Port=66  OutDataTypeStr=int8  PortDimensions=2  VectorParamsAs1DForOutWhenUnconnected=off
  PPort_35_1 : Outport  Port=67  OutDataTypeStr=int8  PortDimensions=2  VectorParamsAs1DForOutWhenUnconnected=off
  PPort_35_2 : Outport  Port=68  OutDataTypeStr=int8  PortDimensions=2  VectorParamsAs1DForOutWhenUnconnected=off
  PPort_36_1 : Outport  Port=69  OutDataTypeStr=int8  PortDimensions=2  VectorParamsAs1DForOutWhenUnconnected=off
  PPort_36_2 : Outport  Port=70  OutDataTypeStr=int8  PortDimensions=2  VectorParamsAs1DForOutWhenUnconnected=off
  PPort_37_1 : Outport  Port=71  OutDataTypeStr=int8  PortDimensions=2  VectorParamsAs1DForOutWhenUnconnected=off
  PPort_37_2 : Outport  Port=72  OutDataTypeStr=int8  PortDimensions=2  VectorParamsAs1DForOutWhenUnconnected=off
  PPort_38_1 : Outport  Port=73  OutDataTypeStr=int8  PortDimensions=2  VectorParamsAs1DForOutWhenUnconnected=off
  PPort_38_2 : Outport  Port=74  OutDataTypeStr=int8  PortDimensions=2  VectorParamsAs1DForOutWhenUnconnected=off
  PPort_39_1 : Outport  Port=75  OutDataTypeStr=int8  PortDimensions=2  VectorParamsAs1DForOutWhenUnconnected=off
  PPort_39_2 : Outport  Port=76  OutDataTypeStr=int8  PortDimensions=2  VectorParamsAs1DForOutWhenUnconnected=off
  PPort_40_1 : Outport  Port=77  OutDataTypeStr=int8  PortDimensions=2  VectorParamsAs1DForOutWhenUnconnected=off
  PPort_40_2 : Outport  Port=78  OutDataTypeStr=int8  PortDimensions=2  VectorParamsAs1DForOutWhenUnconnected=off
  PPort_41_1 : Outport  Port=79  OutDataTypeStr=int8  PortDimensions=2  VectorParamsAs1DForOutWhenUnconnected=off
  PPort_41_2 : Outport  Port=80  OutDataTypeStr=int8  PortDimensions=2  VectorParamsAs1DForOutWhenUnconnected=off
  PPort_42_1 : Outport  Port=81  OutDataTypeStr=int8  PortDimensions=2  VectorParamsAs1DForOutWhenUnconnected=off
  PPort_42_2 : Outport  Port=82  OutDataTypeStr=int8  PortDimensions=2  VectorParamsAs1DForOutWhenUnconnected=off
  PPort_43_1 : Outport  Port=83  OutDataTypeStr=int8  PortDimensions=2  VectorParamsAs1DForOutWhenUnconnected=off
  PPort_43_2 : Outport  Port=84  OutDataTypeStr=int8  PortDimensions=2  VectorParamsAs1DForOutWhenUnconnected=off
  PPort_44_1 : Outport  Port=85  OutDataTypeStr=int8  PortDimensions=2  VectorParamsAs1DForOutWhenUnconnected=off
  PPort_44_2 : Outport  Port=86  OutDataTypeStr=int8  PortDimensions=2  VectorParamsAs1DForOutWhenUnconnected=off
  PPort_45_1 : Outport  Port=87  OutDataTypeStr=int8  PortDimensions=2  VectorParamsAs1DForOutWhenUnconnected=off
  PPort_45_2 : Outport  Port=88  OutDataTypeStr=int8  PortDimensions=2  VectorParamsAs1DForOutWhenUnconnected=off
  PPort_46_1 : Outport  Port=89  OutDataTypeStr=int8  PortDimensions=2  VectorParamsAs1DForOutWhenUnconnected=off
  PPort_46_2 : Outport  Port=90  OutDataTypeStr=int8  PortDimensions=2  VectorParamsAs1DForOutWhenUnconnected=off
  PPort_47_1 : Outport  Port=91  OutDataTypeStr=int8  PortDimensions=2  VectorParamsAs1DForOutWhenUnconnected=off
  PPort_47_2 : Outport  Port=92  OutDataTypeStr=int8  PortDimensions=2  VectorParamsAs1DForOutWhenUnconnected=off
  PPort_48_1 : Outport  Port=93  OutDataTypeStr=int8  PortDimensions=2  VectorParamsAs1DForOutWhenUnconnected=off
  PPort_48_2 : Outport  Port=94  OutDataTypeStr=int8  PortDimensions=2  VectorParamsAs1DForOutWhenUnconnected=off
  PPort_49_1 : Outport  Port=95  OutDataTypeStr=int8  PortDimensions=2  VectorParamsAs1DForOutWhenUnconnected=off
  PPort_49_2 : Outport  Port=96  OutDataTypeStr=int8  PortDimensions=2  VectorParamsAs1DForOutWhenUnconnected=off
  PPort_50_1 : Outport  Port=97  OutDataTypeStr=int8  PortDimensions=2  VectorParamsAs1DForOutWhenUnconnected=off
  PPort_50_2 : Outport  Port=98  OutDataTypeStr=int8  PortDimensions=2  VectorParamsAs1DForOutWhenUnconnected=off
  PPort_51_1 : Outport  Port=99  OutDataTypeStr=int8  PortDimensions=2  VectorParamsAs1DForOutWhenUnconnected=off
  PPort_51_2 : Outport  Port=100  OutDataTypeStr=int8  PortDimensions=2  VectorParamsAs1DForOutWhenUnconnected=off
  PPort_52_1 : Outport  Port=101  OutDataTypeStr=int8  PortDimensions=2  VectorParamsAs1DForOutWhenUnconnected=off
  PPort_52_2 : Outport  Port=102  OutDataTypeStr=int8  PortDimensions=2  VectorParamsAs1DForOutWhenUnconnected=off
  PPort_53_1 : Outport  Port=103  OutDataTypeStr=int8  PortDimensions=2  VectorParamsAs1DForOutWhenUnconnected=off
  PPort_53_2 : Outport  Port=104  OutDataTypeStr=int8  PortDimensions=2  VectorParamsAs1DForOutWhenUnconnected=off
  PPort_54_1 : Outport  Port=105  OutDataTypeStr=int8  PortDimensions=2  VectorParamsAs1DForOutWhenUnconnected=off
  PPort_54_2 : Outport  Port=106  OutDataTypeStr=int8  PortDimensions=2  VectorParamsAs1DForOutWhenUnconnected=off
  PPort_55_1 : Outport  Port=107  OutDataTypeStr=int8  PortDimensions=2  VectorParamsAs1DForOutWhenUnconnected=off
  PPort_55_2 : Outport  Port=108  OutDataTypeStr=int8  PortDimensions=2  VectorParamsAs1DForOutWhenUnconnected=off
  PPort_56_1 : Outport  Port=109  OutDataTypeStr=int8  PortDimensions=2  VectorParamsAs1DForOutWhenUnconnected=off
  PPort_56_2 : Outport  Port=110  OutDataTypeStr=int8  PortDimensions=2  VectorParamsAs1DForOutWhenUnconnected=off
  PPort_57_1 : Outport  Port=111  OutDataTypeStr=int8  PortDimensions=2  VectorParamsAs1DForOutWhenUnconnected=off
  PPort_57_2 : Outport  Port=112  OutDataTypeStr=int8  PortDimensions=2  VectorParamsAs1DForOutWhenUnconnected=off
  PPort_58_1 : Outport  Port=113  OutDataTypeStr=int8  PortDimensions=2  VectorParamsAs1DForOutWhenUnconnected=off
  PPort_58_2 : Outport  Port=114  OutDataTypeStr=int8  PortDimensions=2  VectorParamsAs1DForOutWhenUnconnected=off
  PPort_59_1 : Outport  Port=115  OutDataTypeStr=int8  PortDimensions=2  VectorParamsAs1DForOutWhenUnconnected=off
  PPort_59_2 : Outport  Port=116  OutDataTypeStr=int8  PortDimensions=2  VectorParamsAs1DForOutWhenUnconnected=off
  PPort_60_1 : Outport  Port=117  OutDataTypeStr=int8  PortDimensions=2  VectorParamsAs1DForOutWhenUnconnected=off
  PPort_60_2 : Outport  Port=118  OutDataTypeStr=int8  PortDimensions=2  VectorParamsAs1DForOutWhenUnconnected=off
  PPort_61_1 : Outport  Port=119  OutDataTypeStr=int8  PortDimensions=2  VectorParamsAs1DForOutWhenUnconnected=off
  PPort_61_2 : Outport  Port=120  OutDataTypeStr=int8  PortDimensions=2  VectorParamsAs1DForOutWhenUnconnected=off
  PPort_62_1 : Outport  Port=121  OutDataTypeStr=int8  PortDimensions=2  VectorParamsAs1DForOutWhenUnconnected=off
  PPort_62_2 : Outport  Port=122  OutDataTypeStr=int8  PortDimensions=2  VectorParamsAs1DForOutWhenUnconnected=off
  PPort_63_1 : Outport  Port=123  OutDataTypeStr=int8  PortDimensions=2  VectorParamsAs1DForOutWhenUnconnected=off
  PPort_63_2 : Outport  Port=124  OutDataTypeStr=int8  PortDimensions=2  VectorParamsAs1DForOutWhenUnconnected=off
  PPort_64_1 : Outport  Port=125  OutDataTypeStr=int8  PortDimensions=2  VectorParamsAs1DForOutWhenUnconnected=off
  PPort_64_2 : Outport  Port=126  OutDataTypeStr=int8  PortDimensions=2  VectorParamsAs1DForOutWhenUnconnected=off
  PPort_65_1 : Outport  Port=127  OutDataTypeStr=int8  PortDimensions=2  VectorParamsAs1DForOutWhenUnconnected=off
  PPort_65_2 : Outport  Port=128  OutDataTypeStr=int8  PortDimensions=2  VectorParamsAs1DForOutWhenUnconnected=off
  PPort_66_1 : Outport  Port=129  OutDataTypeStr=int8  PortDimensions=2  VectorParamsAs1DForOutWhenUnconnected=off
  PPort_66_2 : Outport  Port=130  OutDataTypeStr=int8  PortDimensions=2  VectorParamsAs1DForOutWhenUnconnected=off
  PPort_67_1 : Outport  Port=131  OutDataTypeStr=int8  PortDimensions=2  VectorParamsAs1DForOutWhenUnconnected=off
  PPort_67_2 : Outport  Port=132  OutDataTypeStr=int8  PortDimensions=2  VectorParamsAs1DForOutWhenUnconnected=off
  PPort_68_1 : Outport  Port=133  OutDataTypeStr=int8  PortDimensions=2  VectorParamsAs1DForOutWhenUnconnected=off
  PPort_68_2 : Outport  Port=134  OutDataTypeStr=int8  PortDimensions=2  VectorParamsAs1DForOutWhenUnconnected=off
  PPort_69_1 : Outport  Port=135  OutDataTypeStr=int8  PortDimensions=2  VectorParamsAs1DForOutWhenUnconnected=off
  PPort_69_2 : Outport  Port=136  OutDataTypeStr=int8  PortDimensions=2  VectorParamsAs1DForOutWhenUnconnected=off
  PPort_70_1 : Outport  Port=137  OutDataTypeStr=int8  PortDimensions=2  VectorParamsAs1DForOutWhenUnconnected=off
  PPort_70_2 : Outport  Port=138  OutDataTypeStr=int8  PortDimensions=2  VectorParamsAs1DForOutWhenUnconnected=off
  PPort_71_1 : Outport  Port=139  OutDataTypeStr=int8  PortDimensions=2  VectorParamsAs1DForOutWhenUnconnected=off
  PPort_71_2 : Outport  Port=140  OutDataTypeStr=int8  PortDimensions=2  VectorParamsAs1DForOutWhenUnconnected=off
  PPort_72_1 : Outport  Port=141  OutDataTypeStr=int8  PortDimensions=2  VectorParamsAs1DForOutWhenUnconnected=off
  PPort_72_2 : Outport  Port=142  OutDataTypeStr=int8  PortDimensions=2  VectorParamsAs1DForOutWhenUnconnected=off
  PPort_73_1 : Outport  Port=143  OutDataTypeStr=int8  PortDimensions=2  VectorParamsAs1DForOutWhenUnconnected=off
  PPort_73_2 : Outport  Port=144  OutDataTypeStr=int8  PortDimensions=2  VectorParamsAs1DForOutWhenUnconnected=off
  PPort_74_1 : Outport  Port=145  OutDataTypeStr=int8  PortDimensions=2  VectorParamsAs1DForOutWhenUnconnected=off
  PPort_74_2 : Outport  Port=146  OutDataTypeStr=int8  PortDimensions=2  VectorParamsAs1DForOutWhenUnconnected=off
  PPort_75_1 : Outport  Port=147  OutDataTypeStr=int8  PortDimensions=2  VectorParamsAs1DForOutWhenUnconnected=off
  PPort_76_1 : Outport  Port=148  OutDataTypeStr=int8  PortDimensions=2  VectorParamsAs1DForOutWhenUnconnected=off
  PPort_76_2 : Outport  Port=149  OutDataTypeStr=int8  PortDimensions=2  VectorParamsAs1DForOutWhenUnconnected=off
  PPort_77_1 : Outport  Port=150  OutDataTypeStr=int8  PortDimensions=2  VectorParamsAs1DForOutWhenUnconnected=off
  PPort_77_2 : Outport  Port=151  OutDataTypeStr=int8  PortDimensions=2  VectorParamsAs1DForOutWhenUnconnected=off
  PPort_78_1 : Outport  Port=152  OutDataTypeStr=int8  PortDimensions=2  VectorParamsAs1DForOutWhenUnconnected=off
  PPort_78_2 : Outport  Port=153  OutDataTypeStr=int8  PortDimensions=2  VectorParamsAs1DForOutWhenUnconnected=off
  PPort_79_1 : Outport  Port=154  OutDataTypeStr=int8  PortDimensions=2  VectorParamsAs1DForOutWhenUnconnected=off
  PPort_79_2 : Outport  Port=155  OutDataTypeStr=int8  PortDimensions=2  VectorParamsAs1DForOutWhenUnconnected=off
  PPort_80_1 : Outport  Port=156  OutDataTypeStr=int8  PortDimensions=2  VectorParamsAs1DForOutWhenUnconnected=off
  PPort_80_2 : Outport  Port=157  OutDataTypeStr=int8  PortDimensions=2  VectorParamsAs1DForOutWhenUnconnected=off
  PPort_81_1 : Outport  Port=158  OutDataTypeStr=int8  PortDimensions=2  VectorParamsAs1DForOutWhenUnconnected=off
  PPort_81_2 : Outport  Port=159  OutDataTypeStr=int8  PortDimensions=2  VectorParamsAs1DForOutWhenUnconnected=off
  PPort_82_1 : Outport  Port=160  OutDataTypeStr=int8  PortDimensions=2  VectorParamsAs1DForOutWhenUnconnected=off
  PPort_82_2 : Outport  Port=161  OutDataTypeStr=int8  PortDimensions=2  VectorParamsAs1DForOutWhenUnconnected=off
  PPort_83_1 : Outport  Port=162  OutDataTypeStr=int8  PortDimensions=2  VectorParamsAs1DForOutWhenUnconnected=off
  PPort_83_2 : Outport  Port=163  OutDataTypeStr=int8  PortDimensions=2  VectorParamsAs1DForOutWhenUnconnected=off
  PPort_84_1 : Outport  Port=164  OutDataTypeStr=int8  PortDimensions=2  VectorParamsAs1DForOutWhenUnconnected=off
  PPort_84_2 : Outport  Port=165  OutDataTypeStr=int8  PortDimensions=2  VectorParamsAs1DForOutWhenUnconnected=off
  PPort_85_1 : Outport  Port=166  OutDataTypeStr=int8  PortDimensions=2  VectorParamsAs1DForOutWhenUnconnected=off
  PPort_85_2 : Outport  Port=167  OutDataTypeStr=int8  PortDimensions=2  VectorParamsAs1DForOutWhenUnconnected=off
  PPort_86_1 : Outport  Port=168  OutDataTypeStr=int8  PortDimensions=2  VectorParamsAs1DForOutWhenUnconnected=off
  PPort_86_2 : Outport  Port=169  OutDataTypeStr=int8  PortDimensions=2  VectorParamsAs1DForOutWhenUnconnected=off
  PPort_87_1 : Outport  Port=170  OutDataTypeStr=int8  PortDimensions=2  VectorParamsAs1DForOutWhenUnconnected=off
  PPort_87_2 : Outport  Port=171  OutDataTypeStr=int8  PortDimensions=2  VectorParamsAs1DForOutWhenUnconnected=off
  PPort_88_1 : Outport  Port=172  OutDataTypeStr=int8  PortDimensions=2  VectorParamsAs1DForOutWhenUnconnected=off
  PPort_88_2 : Outport  Port=173  OutDataTypeStr=int8  PortDimensions=2  VectorParamsAs1DForOutWhenUnconnected=off
  PPort_89_1 : Outport  Port=174  OutDataTypeStr=int8  PortDimensions=2  VectorParamsAs1DForOutWhenUnconnected=off
  PPort_89_2 : Outport  Port=175  OutDataTypeStr=int8  PortDimensions=2  VectorParamsAs1DForOutWhenUnconnected=off
  PPort_90_1 : Outport  Port=176  OutDataTypeStr=int8  PortDimensions=2  VectorParamsAs1DForOutWhenUnconnected=off
  PPort_90_2 : Outport  Port=177  OutDataTypeStr=int8  PortDimensions=2  VectorParamsAs1DForOutWhenUnconnected=off
  PPort_91_1 : Outport  Port=178  OutDataTypeStr=int8  PortDimensions=2  VectorParamsAs1DForOutWhenUnconnected=off
  PPort_91_2 : Outport  Port=179  OutDataTypeStr=int8  PortDimensions=2  VectorParamsAs1DForOutWhenUnconnected=off
  PPort_92_1 : Outport  Port=180  OutDataTypeStr=int8  PortDimensions=2  VectorParamsAs1DForOutWhenUnconnected=off
  PPort_92_2 : Outport  Port=181  OutDataTypeStr=int8  PortDimensions=2  VectorParamsAs1DForOutWhenUnconnected=off
  PPort_93_1 : Outport  Port=182  OutDataTypeStr=int8  PortDimensions=2  VectorParamsAs1DForOutWhenUnconnected=off
  PPort_93_2 : Outport  Port=183  OutDataTypeStr=int8  PortDimensions=2  VectorParamsAs1DForOutWhenUnconnected=off
  PPort_94_1 : Outport  Port=184  OutDataTypeStr=int8  PortDimensions=2  VectorParamsAs1DForOutWhenUnconnected=off
  PPort_94_2 : Outport  Port=185  OutDataTypeStr=int8  PortDimensions=2  VectorParamsAs1DForOutWhenUnconnected=off
  PPort_95_1 : Outport  Port=186  OutDataTypeStr=int8  PortDimensions=2  VectorParamsAs1DForOutWhenUnconnected=off
  PPort_95_2 : Outport  Port=187  OutDataTypeStr=int8  PortDimensions=2  VectorParamsAs1DForOutWhenUnconnected=off
  PPort_96_1 : Outport  Port=188  OutDataTypeStr=int8  PortDimensions=2  VectorParamsAs1DForOutWhenUnconnected=off
  PPort_96_2 : Outport  Port=189  OutDataTypeStr=int8  PortDimensions=2  VectorParamsAs1DForOutWhenUnconnected=off
  PPort_97_1 : Outport  Port=190  OutDataTypeStr=int8  PortDimensions=2  VectorParamsAs1DForOutWhenUnconnected=off
  PPort_97_2 : Outport  Port=191  OutDataTypeStr=int8  PortDimensions=2  VectorParamsAs1DForOutWhenUnconnected=off
  PPort_98_1 : Outport  Port=192  OutDataTypeStr=int8  PortDimensions=2  VectorParamsAs1DForOutWhenUnconnected=off
  PPort_98_2 : Outport  Port=193  OutDataTypeStr=int8  PortDimensions=2  VectorParamsAs1DForOutWhenUnconnected=off
  PPort_99_1 : Outport  Port=194  OutDataTypeStr=int8  PortDimensions=2  VectorParamsAs1DForOutWhenUnconnected=off
  PPort_99_2 : Outport  Port=195  OutDataTypeStr=int8  PortDimensions=2  VectorParamsAs1DForOutWhenUnconnected=off
  PPort_100_1 : Outport  Port=196  OutDataTypeStr=int8  PortDimensions=2  VectorParamsAs1DForOutWhenUnconnected=off
  PPort_100_2 : Outport  Port=197  OutDataTypeStr=int8  PortDimensions=2  VectorParamsAs1DForOutWhenUnconnected=off
  PPort_101_1 : Outport  Port=198  OutDataTypeStr=int8  PortDimensions=2  VectorParamsAs1DForOutWhenUnconnected=off
  PPort_101_2 : Outport  Port=199  OutDataTypeStr=int8  PortDimensions=2  VectorParamsAs1DForOutWhenUnconnected=off
  PPort_102_1 : Outport  Port=200  OutDataTypeStr=int8  PortDimensions=2  VectorParamsAs1DForOutWhenUnconnected=off
  PPort_102_2 : Outport  Port=201  OutDataTypeStr=int8  PortDimensions=2  VectorParamsAs1DForOutWhenUnconnected=off
  PPort_103_1 : Outport  Port=202  OutDataTypeStr=int8  PortDimensions=2  VectorParamsAs1DForOutWhenUnconnected=off
  PPort_103_2 : Outport  Port=203  OutDataTypeStr=int8  PortDimensions=2  VectorParamsAs1DForOutWhenUnconnected=off
  PPort_104_1 : Outport  Port=204  OutDataTypeStr=int8  PortDimensions=2  VectorParamsAs1DForOutWhenUnconnected=off
  PPort_104_2 : Outport  Port=205  OutDataTypeStr=int8  PortDimensions=2  VectorParamsAs1DForOutWhenUnconnected=off
  PPort_105_1 : Outport  Port=206  OutDataTypeStr=int8  PortDimensions=2  VectorParamsAs1DForOutWhenUnconnected=off
  PPort_105_2 : Outport  Port=207  OutDataTypeStr=int8  PortDimensions=2  VectorParamsAs1DForOutWhenUnconnected=off
  PPort_106_1 : Outport  Port=208  OutDataTypeStr=int8  PortDimensions=2  VectorParamsAs1DForOutWhenUnconnected=off
  PPort_106_2 : Outport  Port=209  OutDataTypeStr=int8  PortDimensions=2  VectorParamsAs1DForOutWhenUnconnected=off
  PPort_107_1 : Outport  Port=210  OutDataTypeStr=int8  PortDimensions=2  VectorParamsAs1DForOutWhenUnconnected=off
  PPort_107_2 : Outport  Port=211  OutDataTypeStr=int8  PortDimensions=2  VectorParamsAs1DForOutWhenUnconnected=off
  PPort_108_1 : Outport  Port=212  OutDataTypeStr=int8  PortDimensions=2  VectorParamsAs1DForOutWhenUnconnected=off
  PPort_108_2 : Outport  Port=213  OutDataTypeStr=int8  PortDimensions=2  VectorParamsAs1DForOutWhenUnconnected=off
  PPort_75_2 : Outport  Port=214  OutDataTypeStr=int8  PortDimensions=2  VectorParamsAs1DForOutWhenUnconnected=off
  wires:
  [B] -> Runnable1_subsystem/3(In2)  "irv3"
  Runnable3_subsystem/1(TicToc_irv) -> [B]
  [A] -> Runnable2_subsystem/2(In2)
  Runnable3_subsystem/3(Multiplier) -> [A]  "irv2"
  RPort_DE1_ErrorStatus/1 -> Runnable1_subsystem/2(ErrorStatus)
  Runnable2_subsystem/2(Subtracter) -> Scope3/1, PPort_DE4/1  "PPort_DE4"
  RPort_DE1/1 -> Runnable1_subsystem/1(In1)
  Runnable2/1 -> Runnable2_subsystem/Trigger
  Runnable1_subsystem/1(TicToc) -> Scope1/1, PPort_DE1/1  "PPort_DE1"
  Runnable2_subsystem/1(TicToc) -> Scope2/1, PPort_DE3/1, Runnable4_subsystem/1(u)  "PPort_DE3"
  Runnable3_subsystem/2(TicToc) -> Scope3/2, PPort_DE2/1  "PPort_DE2"
  Runnable1/1 -> Runnable1_subsystem/Trigger
  Runnable1_subsystem/2(Adder) -> Runnable2_subsystem/1(In1)  "irv1"
  Runnable2_subsystem/3(Subtracter_irv) -> Runnable3_subsystem/1(In1)  "irv4"
  RPort_DE2/1 -> Runnable3_subsystem/2(In2)
  Runnable3/1 -> Runnable3_subsystem/Trigger
  Runnable4/1 -> Runnable4_subsystem/Trigger
  Runnable4_subsystem/1(y) -> Runnable5_subsystem/1(u), PPort_4_1/1  "irv6"
  Runnable4_subsystem/2(y1) -> PPort_4_2/1
  Runnable5_subsystem/1(y) -> Runnable6_subsystem/1(u), PPort_5_1/1  "irv7"
  Runnable5/1 -> Runnable5_subsystem/Trigger
  Runnable5_subsystem/2(y1) -> PPort_5_2/1
  Runnable6_subsystem/2(y1) -> PPort_6_2/1
  Runnable6/1 -> Runnable6_subsystem/Trigger
  Runnable6_subsystem/1(y) -> Runnable7_subsystem/1(u), PPort_6_1/1  "irv8"
  Runnable7_subsystem/2(y1) -> PPort_7_2/1
  Runnable7_subsystem/1(y) -> Runnable8_subsystem/1(u), PPort_7_1/1  "irv9"
  Runnable7/1 -> Runnable7_subsystem/Trigger
  Runnable8_subsystem/2(y1) -> PPort_8_2/1
  Runnable8/1 -> Runnable8_subsystem/Trigger
  Runnable8_subsystem/1(y) -> Runnable9_subsystem/1(u), PPort_8_1/1  "irv10"
  Runnable9_subsystem/1(y) -> Runnable10_subsystem/1(u), PPort_9_1/1  "irv11"
  Runnable9/1 -> Runnable9_subsystem/Trigger
  Runnable9_subsystem/2(y1) -> PPort_9_2/1
  Runnable10_subsystem/2(y1) -> PPort_10_2/1
  Runnable10_subsystem/1(y) -> Runnable11_subsystem/1(u), PPort_10_1/1  "irv12"
  Runnable10/1 -> Runnable10_subsystem/Trigger
  Runnable11/1 -> Runnable11_subsystem/Trigger
  Runnable11_subsystem/1(y) -> Runnable12_subsystem/1(u), PPort_11_1/1  "irv13"
  Runnable11_subsystem/2(y1) -> PPort_11_2/1
  Runnable12_subsystem/1(y) -> Runnable13_subsystem/1(u), PPort_12_1/1  "irv14"
  Runnable12_subsystem/2(y1) -> PPort_12_2/1
  Runnable12/1 -> Runnable12_subsystem/Trigger
  Runnable13/1 -> Runnable13_subsystem/Trigger
  Runnable13_subsystem/2(y1) -> PPort_13_2/1
  Runnable13_subsystem/1(y) -> Runnable14_subsystem/1(u), PPort_13_1/1  "irv15"
  Runnable14/1 -> Runnable14_subsystem/Trigger
  Runnable14_subsystem/2(y1) -> PPort_14_2/1
  Runnable14_subsystem/1(y) -> Runnable15_subsystem/1(u), PPort_14_1/1  "irv16"
  Runnable15_subsystem/1(y) -> Runnable16_subsystem/1(u), PPort_15_1/1  "irv17"
  Runnable15_subsystem/2(y1) -> PPort_15_2/1
  Runnable15/1 -> Runnable15_subsystem/Trigger
  Runnable16_subsystem/1(y) -> Runnable17_subsystem/1(u), PPort_16_1/1  "irv18"
  Runnable16_subsystem/2(y1) -> PPort_16_2/1
  Runnable16/1 -> Runnable16_subsystem/Trigger
  Runnable17_subsystem/1(y) -> Runnable18_subsystem/1(u), PPort_17_1/1  "irv19"
  Runnable17_subsystem/2(y1) -> PPort_17_2/1
  Runnable17/1 -> Runnable17_subsystem/Trigger
  Runnable18/1 -> Runnable18_subsystem/Trigger
  Runnable18_subsystem/2(y1) -> PPort_18_2/1
  Runnable18_subsystem/1(y) -> Runnable19_subsystem/1(u), PPort_18_1/1  "irv20"
  Runnable19_subsystem/1(y) -> Runnable20_subsystem/1(u), PPort_19_1/1  "irv21"
  Runnable19_subsystem/2(y1) -> PPort_19_2/1
  Runnable19/1 -> Runnable19_subsystem/Trigger
  Runnable20/1 -> Runnable20_subsystem/Trigger
  Runnable20_subsystem/1(y) -> Runnable21_subsystem/1(u), PPort_20_1/1  "irv22"
  Runnable20_subsystem/2(y1) -> PPort_20_2/1
  Runnable21_subsystem/2(y1) -> PPort_21_2/1
  Runnable21_subsystem/1(y) -> Runnable22_subsystem/1(u), PPort_21_1/1  "irv23"
  Runnable21/1 -> Runnable21_subsystem/Trigger
  Runnable22_subsystem/2(y1) -> PPort_22_2/1
  Runnable22_subsystem/1(y) -> Runnable23_subsystem/1(u), PPort_22_1/1  "irv24"
  Runnable22/1 -> Runnable22_subsystem/Trigger
  Runnable23_subsystem/2(y1) -> PPort_23_2/1
  Runnable23_subsystem/1(y) -> Runnable24_subsystem/1(u), PPort_23_1/1  "irv25"
  Runnable23/1 -> Runnable23_subsystem/Trigger
  Runnable24_subsystem/2(y1) -> PPort_24_2/1
  Runnable24_subsystem/1(y) -> Runnable25_subsystem/1(u), PPort_24_1/1  "irv26"
  Runnable24/1 -> Runnable24_subsystem/Trigger
  Runnable25_subsystem/2(y1) -> PPort_25_2/1
  Runnable25_subsystem/1(y) -> Runnable26_subsystem/1(u), PPort_25_1/1  "irv27"
  Runnable25/1 -> Runnable25_subsystem/Trigger
  Runnable26_subsystem/2(y1) -> PPort_26_2/1
  Runnable26_subsystem/1(y) -> Runnable27_subsystem/1(u), PPort_26_1/1  "irv28"
  Runnable26/1 -> Runnable26_subsystem/Trigger
  Runnable27_subsystem/2(y1) -> PPort_27_2/1
  Runnable27_subsystem/1(y) -> Runnable28_subsystem/1(u), PPort_27_1/1  "irv29"
  Runnable27/1 -> Runnable27_subsystem/Trigger
  Runnable28_subsystem/2(y1) -> PPort_28_2/1
  Runnable28_subsystem/1(y) -> Runnable29_subsystem/1(u), PPort_28_1/1  "irv30"
  Runnable28/1 -> Runnable28_subsystem/Trigger
  Runnable29_subsystem/2(y1) -> PPort_29_2/1
  Runnable29/1 -> Runnable29_subsystem/Trigger
  Runnable30_subsystem/2(y1) -> PPort_30_2/1
  Runnable30_subsystem/1(y) -> Runnable31_subsystem/1(u), PPort_30_1/1  "irv32"
  Runnable30/1 -> Runnable30_subsystem/Trigger
  Runnable31_subsystem/2(y1) -> PPort_31_2/1
  Runnable31_subsystem/1(y) -> Runnable32_subsystem/1(u), PPort_31_1/1  "irv33"
  Runnable31/1 -> Runnable31_subsystem/Trigger
  Runnable32_subsystem/2(y1) -> PPort_32_2/1
  Runnable32_subsystem/1(y) -> Runnable33_subsystem/1(u), PPort_32_1/1  "irv34"
  Runnable32/1 -> Runnable32_subsystem/Trigger
  Runnable33_subsystem/2(y1) -> PPort_33_2/1
  Runnable33/1 -> Runnable33_subsystem/Trigger
  Runnable34_subsystem/2(y1) -> PPort_34_2/1
  Runnable34_subsystem/1(y) -> Runnable35_subsystem/1(u), PPort_34_1/1  "irv36"
  Runnable34/1 -> Runnable34_subsystem/Trigger
  Runnable35_subsystem/2(y1) -> PPort_35_2/1
  Runnable35_subsystem/1(y) -> Runnable36_subsystem/1(u), PPort_35_1/1  "irv37"
  Runnable35/1 -> Runnable35_subsystem/Trigger
  Runnable36_subsystem/2(y1) -> PPort_36_2/1
  Runnable36_subsystem/1(y) -> Runnable37_subsystem/1(u), PPort_36_1/1  "irv38"
  Runnable36/1 -> Runnable36_subsystem/Trigger
  Runnable37_subsystem/2(y1) -> PPort_37_2/1
  Runnable37_subsystem/1(y) -> Runnable38_subsystem/1(u), PPort_37_1/1  "irv39"
  Runnable37/1 -> Runnable37_subsystem/Trigger
  Runnable38_subsystem/2(y1) -> PPort_38_2/1
  Runnable38_subsystem/1(y) -> Runnable39_subsystem/1(u), PPort_38_1/1  "irv40"
  Runnable38/1 -> Runnable38_subsystem/Trigger
  Runnable39_subsystem/2(y1) -> PPort_39_2/1
  Runnable39_subsystem/1(y) -> Runnable40_subsystem/1(u), PPort_39_1/1  "irv41"
  Runnable39/1 -> Runnable39_subsystem/Trigger
  Runnable40_subsystem/2(y1) -> PPort_40_2/1
  Runnable40_subsystem/1(y) -> Runnable41_subsystem/1(u), PPort_40_1/1  "irv42"
  Runnable40/1 -> Runnable40_subsystem/Trigger
  Runnable46/1 -> Runnable46_subsystem/Trigger
  Runnable46_subsystem/1(y) -> Runnable47_subsystem/1(u), PPort_46_1/1  "irv48"
  Runnable43_subsystem/2(y1) -> PPort_43_2/1
  Runnable43/1 -> Runnable43_subsystem/Trigger
  Runnable43_subsystem/1(y) -> Runnable44_subsystem1/1(u), PPort_43_1/1  "irv45"
  Runnable44_subsystem1/1(y) -> Runnable45_subsystem/1(u), PPort_44_1/1  "irv46"
  Runnable44/1 -> Runnable44_subsystem1/Trigger
  Runnable49_subsystem/1(y) -> Runnable50_subsystem1/1(u), PPort_49_1/1  "irv51"
  Runnable50_subsystem1/1(y) -> Runnable51_subsystem2/1(u), PPort_50_1/1  "irv52"
  Runnable49_subsystem/2(y1) -> PPort_49_2/1
  Runnable50/1 -> Runnable50_subsystem1/Trigger
  Runnable50_subsystem1/2(y1) -> PPort_50_2/1
  Runnable45/1 -> Runnable45_subsystem/Trigger
  Runnable44_subsystem1/2(y1) -> PPort_44_2/1
  Runnable45_subsystem/1(y) -> Runnable46_subsystem/1(u), PPort_45_1/1  "irv47"
  Runnable47/1 -> Runnable47_subsystem/Trigger
  Runnable47_subsystem/2(y1) -> PPort_47_2/1
  Runnable49/1 -> Runnable49_subsystem/Trigger
  Runnable47_subsystem/1(y) -> Runnable48_subsystem/1(u), PPort_47_1/1  "irv49"
  Runnable46_subsystem/2(y1) -> PPort_46_2/1
  Runnable42/1 -> Runnable42_subsystem/Trigger
  Runnable48_subsystem/2(y1) -> PPort_48_2/1
  Runnable42_subsystem/1(y) -> Runnable43_subsystem/1(u), PPort_42_1/1  "irv44"
  Runnable45_subsystem/2(y1) -> PPort_45_2/1
  Runnable41/1 -> Runnable41_subsystem/Trigger
  Runnable41_subsystem/2(y1) -> PPort_41_2/1
  Runnable48_subsystem/1(y) -> Runnable49_subsystem/1(u), PPort_48_1/1  "irv50"
  Runnable48/1 -> Runnable48_subsystem/Trigger
  Runnable42_subsystem/2(y1) -> PPort_42_2/1
  Runnable41_subsystem/1(y) -> Runnable42_subsystem/1(u), PPort_41_1/1  "irv43"
  Runnable56/1 -> Runnable56_subsystem2/Trigger
  Runnable56_subsystem2/1(y) -> Runnable57_subsystem2/1(u), PPort_56_1/1  "irv58"
  Runnable53_subsystem2/2(y1) -> PPort_53_2/1
  Runnable53/1 -> Runnable53_subsystem2/Trigger
  Runnable53_subsystem2/1(y) -> Runnable54_subsystem2/1(u), PPort_53_1/1  "irv55"
  Runnable54_subsystem2/1(y) -> Runnable55_subsystem2/1(u), PPort_54_1/1  "irv56"
  Runnable54/1 -> Runnable54_subsystem2/Trigger
  Runnable59_subsystem2/1(y) -> Runnable60_subsystem2/1(u), PPort_59_1/1  "irv61"
  Runnable60_subsystem2/1(y) -> Runnable61_subsystem/1(u), PPort_60_1/1  "irv62"
  Runnable59_subsystem2/2(y1) -> PPort_59_2/1
  Runnable60/1 -> Runnable60_subsystem2/Trigger
  Runnable60_subsystem2/2(y1) -> PPort_60_2/1
  Runnable55/1 -> Runnable55_subsystem2/Trigger
  Runnable54_subsystem2/2(y1) -> PPort_54_2/1
  Runnable55_subsystem2/1(y) -> Runnable56_subsystem2/1(u), PPort_55_1/1  "irv57"
  Runnable57/1 -> Runnable57_subsystem2/Trigger
  Runnable57_subsystem2/2(y1) -> PPort_57_2/1
  Runnable59/1 -> Runnable59_subsystem2/Trigger
  Runnable57_subsystem2/1(y) -> Runnable58_subsystem2/1(u), PPort_57_1/1  "irv59"
  Runnable56_subsystem2/2(y1) -> PPort_56_2/1
  Runnable52/1 -> Runnable52_subsystem2/Trigger
  Runnable58_subsystem2/2(y1) -> PPort_58_2/1
  Runnable52_subsystem2/1(y) -> Runnable53_subsystem2/1(u), PPort_52_1/1  "irv54"
  Runnable55_subsystem2/2(y1) -> PPort_55_2/1
  Runnable51/1 -> Runnable51_subsystem2/Trigger
  Runnable51_subsystem2/2(y1) -> PPort_51_2/1
  Runnable58_subsystem2/1(y) -> Runnable59_subsystem2/1(u), PPort_58_1/1  "irv60"
  Runnable58/1 -> Runnable58_subsystem2/Trigger
  Runnable52_subsystem2/2(y1) -> PPort_52_2/1
  Runnable51_subsystem2/1(y) -> Runnable52_subsystem2/1(u), PPort_51_1/1  "irv53"
  Runnable66/1 -> Runnable66_subsystem3/Trigger
  Runnable66_subsystem3/1(y) -> Runnable67_subsystem/1(u), PPort_66_1/1  "irv68"
  Runnable63_subsystem/2(y1) -> PPort_63_2/1
  Runnable63/1 -> Runnable63_subsystem/Trigger
  Runnable63_subsystem/1(y) -> Runnable64_subsystem/1(u), PPort_63_1/1  "irv65"
  Runnable64_subsystem/1(y) -> Runnable65_subsystem/1(u), PPort_64_1/1  "irv66"
  Runnable64/1 -> Runnable64_subsystem/Trigger
  Runnable69_subsystem/1(y) -> Runnable70_subsystem/1(u), PPort_69_1/1  "irv71"
  Runnable69_subsystem/2(y1) -> PPort_69_2/1
  Runnable70/1 -> Runnable70_subsystem/Trigger
  Runnable70_subsystem/2(y1) -> PPort_70_2/1
  Runnable65/1 -> Runnable65_subsystem/Trigger
  Runnable64_subsystem/2(y1) -> PPort_64_2/1
  Runnable65_subsystem/1(y) -> Runnable66_subsystem3/1(u), PPort_65_1/1  "irv67"
  Runnable67/1 -> Runnable67_subsystem/Trigger
  Runnable67_subsystem/2(y1) -> PPort_67_2/1
  Runnable69/1 -> Runnable69_subsystem/Trigger
  Runnable67_subsystem/1(y) -> Runnable68_subsystem/1(u), PPort_67_1/1  "irv69"
  Runnable66_subsystem3/2(y1) -> PPort_66_2/1
  Runnable62/1 -> Runnable62_subsystem/Trigger
  Runnable68_subsystem/2(y1) -> PPort_68_2/1
  Runnable62_subsystem/1(y) -> Runnable63_subsystem/1(u), PPort_62_1/1  "irv64"
  Runnable65_subsystem/2(y1) -> PPort_65_2/1
  Runnable61/1 -> Runnable61_subsystem/Trigger
  Runnable61_subsystem/2(y1) -> PPort_61_2/1
  Runnable68_subsystem/1(y) -> PPort_68_1/1, Runnable69_subsystem/1(u)  "irv70"
  Runnable68/1 -> Runnable68_subsystem/Trigger
  Runnable62_subsystem/2(y1) -> PPort_62_2/1
  Runnable61_subsystem/1(y) -> Runnable62_subsystem/1(u), PPort_61_1/1  "irv63"
  Runnable76/1 -> Runnable76_subsystem/Trigger
  Runnable76_subsystem/1(y) -> Runnable77_subsystem/1(u), PPort_76_1/1  "irv78"
  Runnable73_subsystem/2(y1) -> PPort_73_2/1
  Runnable73/1 -> Runnable73_subsystem/Trigger
  Runnable73_subsystem/1(y) -> Runnable74_subsystem/1(u), PPort_73_1/1  "irv75"
  Runnable74_subsystem/1(y) -> Runnable75_subsystem/1(u), PPort_74_1/1  "irv76"
  Runnable74/1 -> Runnable74_subsystem/Trigger
  Runnable79_subsystem/1(y) -> Runnable80_subsystem/1(u), PPort_79_1/1  "irv81"
  Runnable80_subsystem/1(y) -> Runnable81_subsystem/1(u), PPort_80_1/1  "irv82"
  Runnable79_subsystem/2(y1) -> PPort_79_2/1
  Runnable80/1 -> Runnable80_subsystem/Trigger
  Runnable80_subsystem/2(y1) -> PPort_80_2/1
  Runnable75/1 -> Runnable75_subsystem/Trigger
  Runnable74_subsystem/2(y1) -> PPort_74_2/1
  Runnable75_subsystem/1(y) -> Runnable76_subsystem/1(u), PPort_75_1/1  "irv77"
  Runnable77/1 -> Runnable77_subsystem/Trigger
  Runnable77_subsystem/2(y1) -> PPort_77_2/1
  Runnable79/1 -> Runnable79_subsystem/Trigger
  Runnable77_subsystem/1(y) -> Runnable78_subsystem/1(u), PPort_77_1/1  "irv79"
  Runnable76_subsystem/2(y1) -> PPort_76_2/1
  Runnable72/1 -> Runnable72_subsystem/Trigger
  Runnable78_subsystem/2(y1) -> PPort_78_2/1
  Runnable72_subsystem/1(y) -> Runnable73_subsystem/1(u), PPort_72_1/1  "irv74"
  Runnable75_subsystem/2(y1) -> PPort_75_2/1
  Runnable71/1 -> Runnable71_subsystem/Trigger
  Runnable71_subsystem/2(y1) -> PPort_71_2/1
  Runnable78_subsystem/1(y) -> Runnable79_subsystem/1(u), PPort_78_1/1  "irv80"
  Runnable78/1 -> Runnable78_subsystem/Trigger
  Runnable72_subsystem/2(y1) -> PPort_72_2/1
  Runnable71_subsystem/1(y) -> Runnable72_subsystem/1(u), PPort_71_1/1  "irv73"
  Runnable86/1 -> Runnable86_subsystem/Trigger
  Runnable86_subsystem/1(y) -> Runnable87_subsystem/1(u), PPort_86_1/1  "irv88"
  Runnable83_subsystem/2(y1) -> PPort_83_2/1
  Runnable83/1 -> Runnable83_subsystem/Trigger
  Runnable83_subsystem/1(y) -> Runnable84_subsystem/1(u), PPort_83_1/1  "irv85"
  Runnable84_subsystem/1(y) -> Runnable85_subsystem/1(u), PPort_84_1/1  "irv86"
  Runnable84/1 -> Runnable84_subsystem/Trigger
  Runnable89_subsystem/1(y) -> Runnable90_subsystem/1(u), PPort_89_1/1  "irv91"
  Runnable90_subsystem/1(y) -> Runnable91_subsystem/1(u), PPort_90_1/1  "irv92"
  Runnable89_subsystem/2(y1) -> PPort_89_2/1
  Runnable90/1 -> Runnable90_subsystem/Trigger
  Runnable90_subsystem/2(y1) -> PPort_90_2/1
  Runnable85/1 -> Runnable85_subsystem/Trigger
  Runnable84_subsystem/2(y1) -> PPort_84_2/1
  Runnable85_subsystem/1(y) -> Runnable86_subsystem/1(u), PPort_85_1/1  "irv87"
  Runnable87/1 -> Runnable87_subsystem/Trigger
  Runnable87_subsystem/2(y1) -> PPort_87_2/1
  Runnable89/1 -> Runnable89_subsystem/Trigger
  Runnable86_subsystem/2(y1) -> PPort_86_2/1
  Runnable82/1 -> Runnable82_subsystem/Trigger
  Runnable88_subsystem/2(y1) -> PPort_88_2/1
  Runnable82_subsystem/1(y) -> Runnable83_subsystem/1(u), PPort_82_1/1  "irv84"
  Runnable85_subsystem/2(y1) -> PPort_85_2/1
  Runnable81/1 -> Runnable81_subsystem/Trigger
  Runnable81_subsystem/2(y1) -> PPort_81_2/1
  Runnable88_subsystem/1(y) -> Runnable89_subsystem/1(u), PPort_88_1/1  "irv90"
  Runnable88/1 -> Runnable88_subsystem/Trigger
  Runnable82_subsystem/2(y1) -> PPort_82_2/1
  Runnable81_subsystem/1(y) -> Runnable82_subsystem/1(u), PPort_81_1/1  "irv83"
  Runnable96/1 -> Runnable96_subsystem/Trigger
  Runnable96_subsystem/1(y) -> Runnable97_subsystem/1(u), PPort_96_1/1  "irv98"
  Runnable93_subsystem/2(y1) -> PPort_93_2/1
  Runnable93/1 -> Runnable93_subsystem/Trigger
  Runnable93_subsystem/1(y) -> Runnable94_subsystem/1(u), PPort_93_1/1  "irv95"
  Runnable94_subsystem/1(y) -> Runnable95_subsystem/1(u), PPort_94_1/1  "irv96"
  Runnable94/1 -> Runnable94_subsystem/Trigger
  Runnable99_subsystem/1(y) -> Runnable100_subsystem/1(u), PPort_99_1/1  "irv101"
  Runnable100_subsystem/1(y) -> Runnable101_subsystem/1(u), PPort_100_1/1  "irv102"
  Runnable99_subsystem/2(y1) -> PPort_99_2/1
  Runnable100/1 -> Runnable100_subsystem/Trigger
  Runnable100_subsystem/2(y1) -> PPort_100_2/1
  Runnable95/1 -> Runnable95_subsystem/Trigger
  Runnable94_subsystem/2(y1) -> PPort_94_2/1
  Runnable95_subsystem/1(y) -> Runnable96_subsystem/1(u), PPort_95_1/1  "irv97"
  Runnable97/1 -> Runnable97_subsystem/Trigger
  Runnable97_subsystem/2(y1) -> PPort_97_2/1
  Runnable99/1 -> Runnable99_subsystem/Trigger
  Runnable97_subsystem/1(y) -> PPort_97_1/1, Runnable98_subsystem/1(u)  "irv99"
  Runnable96_subsystem/2(y1) -> PPort_96_2/1
  Runnable92/1 -> Runnable92_subsystem6/Trigger
  Runnable98_subsystem/2(y1) -> PPort_98_2/1
  Runnable92_subsystem6/1(y) -> Runnable93_subsystem/1(u), PPort_92_1/1  "irv94"
  Runnable95_subsystem/2(y1) -> PPort_95_2/1
  Runnable91/1 -> Runnable91_subsystem/Trigger
  Runnable91_subsystem/2(y1) -> PPort_91_2/1
  Runnable98_subsystem/1(y) -> Runnable99_subsystem/1(u), PPort_98_1/1  "irv100"
  Runnable98/1 -> Runnable98_subsystem/Trigger
  Runnable92_subsystem6/2(y1) -> PPort_92_2/1
  Runnable91_subsystem/1(y) -> Runnable92_subsystem6/1(u), PPort_91_1/1  "irv93"
  Runnable106/1 -> Runnable106_subsystem/Trigger
  Runnable106_subsystem/1(y) -> Runnable107_subsystem/1(u), PPort_106_1/1  "irv108"
  Runnable103_subsystem/2(y1) -> PPort_103_2/1
  Runnable103/1 -> Runnable103_subsystem/Trigger
  Runnable103_subsystem/1(y) -> Runnable104_subsystem/1(u), PPort_103_1/1  "irv105"
  Runnable104_subsystem/1(y) -> Runnable105_subsystem/1(u), PPort_104_1/1  "irv106"
  Runnable104/1 -> Runnable104_subsystem/Trigger
  Runnable105/1 -> Runnable105_subsystem/Trigger
  Runnable104_subsystem/2(y1) -> PPort_104_2/1
  Runnable105_subsystem/1(y) -> Runnable106_subsystem/1(u), PPort_105_1/1  "irv107"
  Runnable107/1 -> Runnable107_subsystem/Trigger
  Runnable107_subsystem/2(y1) -> PPort_107_2/1
  Runnable107_subsystem/1(y) -> Runnable108_subsystem/1(u), PPort_107_1/1  "irv109"
  Runnable106_subsystem/2(y1) -> PPort_106_2/1
  Runnable102/1 -> Runnable102_subsystem/Trigger
  Runnable108_subsystem/2(y1) -> PPort_108_2/1
  Runnable102_subsystem/1(y) -> Runnable103_subsystem/1(u), PPort_102_1/1  "irv104"
  Runnable105_subsystem/2(y1) -> PPort_105_2/1
  Runnable101/1 -> Runnable101_subsystem/Trigger
  Runnable101_subsystem/2(y1) -> PPort_101_2/1
  Runnable108_subsystem/1(y) -> PPort_108_1/1
  Runnable108/1 -> Runnable108_subsystem/Trigger
  Runnable102_subsystem/2(y1) -> PPort_102_2/1
  Runnable101_subsystem/1(y) -> Runnable102_subsystem/1(u), PPort_101_1/1  "irv103"
  Runnable29_subsystem/1(y) -> Runnable30_subsystem/1(u), PPort_29_1/1  "irv31"
  Runnable33_subsystem/1(y) -> Runnable34_subsystem/1(u), PPort_33_1/1  "irv35"
  Runnable70_subsystem/1(y) -> Runnable71_subsystem/1(u), PPort_70_1/1  "irv72"
  Runnable87_subsystem/1(y) -> Runnable88_subsystem/1(u), PPort_87_1/1  "irv89"
